simulink model "DetectorSincronico"  (R2018a)
settings: Solver=FixedStepAuto  StartTime=0.0  StopTime=10  FixedStep=0.00001  RelTol=1e-3  EnableMultiTasking=on
libraries: simulink_extras x1, simulink x1, powerlib_meascontrol x1
settings Model: Creator=Augusto  LastModifiedBy=Augusto

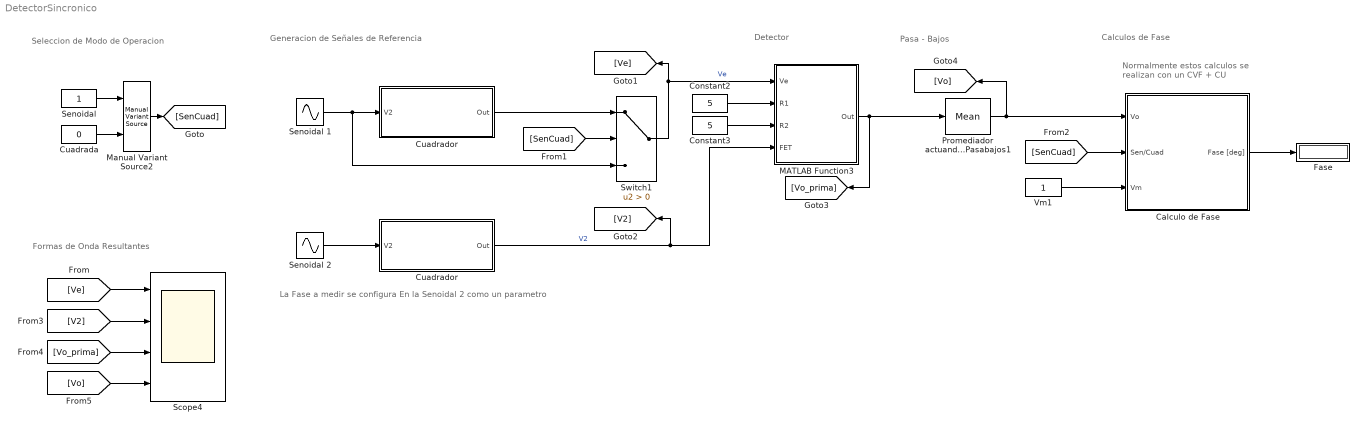
== system DetectorSincronico ==
  note: Normalmente estos calculos se
      | realizan con un CVF + CU
  note: La Fase a medir se configura En la Senoidal 2 como un parametro
  note: Formas de Onda Resultantes
  note: Generacion de Señales de Referencia
  note: Seleccion de Modo de Operacion
  note: Calculos de Fase
  note: Pasa - Bajos
  note: Detector
  Calculo de Fase : Subsystem
  Constant2 : Constant  Value=5
  Constant3 : Constant  Value=5
  Cuadrada : Constant  Value=0
  Cuadrador : MATLAB Function  TreatAsAtomicUnit=on
  "Cuadrador " : MATLAB Function  TreatAsAtomicUnit=on
  Fase : Display
  MATLAB Function3 : MATLAB Function  TreatAsAtomicUnit=on
  Manual Variant Source2 : simulink/Signal Routing/Manual Variant Source  NumChoices=2  OverrideUsingVariant=V_2
      settings: SourceProductName=Simulink
  Promediador actuando como Pasabajos1 : powerlib_meascontrol/Measurements/Mean  Freq=1  Vinit=0  Ts=0
  Scope4 : Scope  NumInputPorts=4
  Senoidal : Constant
  Senoidal 1 : Sin  Frequency=2*pi  SampleTime=0
  Senoidal 2 : Sin  Frequency=2*pi  Phase=(pi/180)*83  SampleTime=0
  Switch1 : Switch  Criteria=u2 > Threshold
  Vm1 : Constant
  wires:
  Promediador actuando como Pasabajos1/1 -> [Vo], Calculo de Fase/1(Vo)
  Constant2/1 -> MATLAB Function3/2(R1)
  Cuadrador/1(Out) -> [V2], MATLAB Function3/4(FET)  "V2"
  Senoidal 2/1 -> Cuadrador/1(V2)
  Senoidal 1/1 -> "Cuadrador "/1(V2), Switch1/3
  Constant3/1 -> MATLAB Function3/3(R2)
  Switch1/1 -> [Ve], MATLAB Function3/1(Ve)  "Ve"
  Vm1/1 -> Calculo de Fase/3(Vm)
  Calculo de Fase/1(Fase [deg]) -> Fase/1
  Senoidal/1 -> Manual Variant Source2/1
  Cuadrada/1 -> Manual Variant Source2/2
  Manual Variant Source2/1 -> [SenCuad]
  [SenCuad] -> Switch1/2
  [SenCuad] -> Calculo de Fase/2(Sen/Cuad)
  "Cuadrador "/1(Out) -> Switch1/1
  MATLAB Function3/1(Out) -> [Vo_prima], Promediador actuando como Pasabajos1/1
  [Ve] -> Scope4/1
  [V2] -> Scope4/2
  [Vo] -> Scope4/4
  [Vo_prima] -> Scope4/3

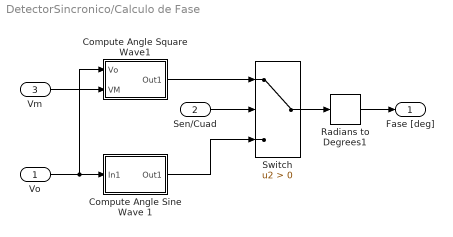
== system DetectorSincronico/Calculo de Fase ==
  Vo : Inport
  Sen/Cuad : Inport  Port=2
  Vm : Inport  Port=3
  Compute Angle Sine Wave 1 : Subsystem
  Compute Angle Square Wave1 : Subsystem
  Radians to Degrees1 : simulink_extras/Transformations/Radians to Degrees
  Switch : Switch  Criteria=u2 > Threshold
  Fase [deg] : Outport
  wires:
  Vm/1 -> Compute Angle Square Wave1/2(VM)
  Switch/1 -> Radians to Degrees1/1
  Radians to Degrees1/1 -> Fase [deg]/1
  Vo/1 -> Compute Angle Square Wave1/1("Vo "), Compute Angle Sine Wave 1/1(In1)
  Sen/Cuad/1 -> Switch/2
  Compute Angle Sine Wave 1/1(Out1) -> Switch/3
  Compute Angle Square Wave1/1(Out1) -> Switch/1

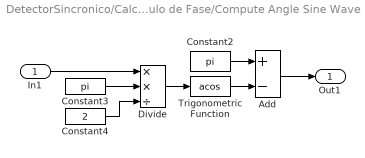
== system DetectorSincronico/Calculo de Fase/Compute Angle Sine Wave 1 ==
  In1 : Inport
  Add : Sum  Inputs=+-
  Constant2 : Constant  Value=pi
  Constant3 : Constant  Value=pi
  Constant4 : Constant  Value=2
  Divide : Product  Inputs=**/
  Trigonometric Function : Trigonometry  Operator=acos
  Out1 : Outport
  wires:
  Constant2/1 -> Add/1
  In1/1 -> Divide/1
  Constant3/1 -> Divide/2
  Divide/1 -> Trigonometric Function/1
  Constant4/1 -> Divide/3
  Trigonometric Function/1 -> Add/2
  Add/1 -> Out1/1

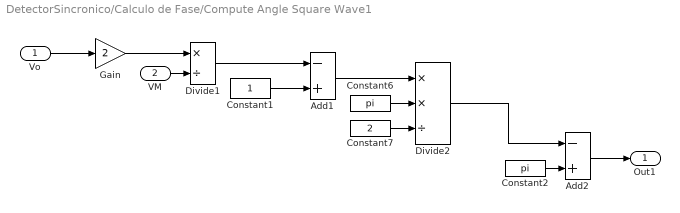
== system DetectorSincronico/Calculo de Fase/Compute Angle Square Wave1 ==
  "Vo " : Inport
  VM : Inport  Port=2
  Add1 : Sum  Inputs=-+
  Add2 : Sum  Inputs=-+
  Constant1 : Constant
  Constant2 : Constant  Value=pi
  Constant6 : Constant  Value=pi
  Constant7 : Constant  Value=2
  Divide1 : Product  Inputs=*/
  Divide2 : Product  Inputs=**/
  Gain : Gain  Gain=2
  Out1 : Outport
  wires:
  "Vo "/1 -> Gain/1
  VM/1 -> Divide1/2
  Divide1/1 -> Add1/1
  Constant1/1 -> Add1/2
  Constant7/1 -> Divide2/3
  Constant6/1 -> Divide2/2
  Add1/1 -> Divide2/1
  Gain/1 -> Divide1/1
  Divide2/1 -> Add2/1
  Add2/1 -> Out1/1
  Constant2/1 -> Add2/2

== matlab function DetectorSincronico/MATLAB Function3 ==
  data: Ve input; Out output; R1 input; R2 input; FET input
function Out = Detector(Ve,R1,R2,FET)
    if FET
        Out = (-R2/R1)*Ve;
    else
        Out = Ve;
    end

== matlab function DetectorSincronico/Cuadrador ==
  data: V2 input; Out output
function Out = CuadradorDeReferencia(V2)
    if V2 >=0
        Out = 1;
    else
        Out = 0;
    end

== matlab function DetectorSincronico/Cuadrador  ==
  data: V2 input; Out output
function Out = CuadradorDeReferencia(V2)
    if V2 >=0
        Out = 1;
    else
        Out = 0;
    end
